simulink model "TD_THRUSTER_M0"  (R2019b)
settings: Solver=FixedStepAuto  StartTime=0.0  StopTime=10.0  RelTol=1e-3
undefined symbols (not defined in the file): w_neg_0, w_pos_0
settings Model: Creator=lbend  LastModifiedBy=peter
settings DebuggingCC: UnconnectedInputMsg=none  UnconnectedOutputMsg=none  UnconnectedLineMsg=none  SFMachineParentedDataDiag=error
settings ModelReferenceCC: EnableRefExpFcnMdlSchedulingChecks=off
settings RTWCC: Description=Generic Real-Time Target

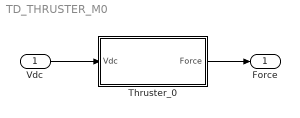
== system TD_THRUSTER_M0 ==
  Vdc : Inport
  Thruster_0 : Subsystem
  Force : Outport
  wires:
  Vdc/1 -> Thruster_0/1(Vdc)
  Thruster_0/1(Force) -> Force/1

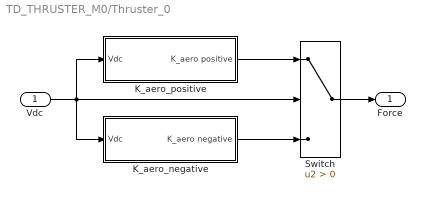
== system TD_THRUSTER_M0/Thruster_0 ==
  Vdc : Inport
  K_aero_negative : Subsystem
  K_aero_positive : Subsystem
  Switch : Switch  Criteria=u2 > Threshold
  Force : Outport
  wires:
  Switch/1 -> Force/1
  K_aero_positive/1(K_aero positive) -> Switch/1
  Vdc/1 -> K_aero_positive/1(Vdc), K_aero_negative/1(Vdc), Switch/2
  K_aero_negative/1(K_aero negative) -> Switch/3

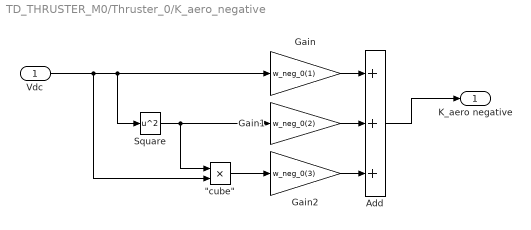
== system TD_THRUSTER_M0/Thruster_0/K_aero_negative ==
  Vdc : Inport
  "\"cube\"" : Product  Inputs=**
  Add : Sum  Inputs=+++
  Gain : Gain  Gain=w_neg_0(1)
  Gain1 : Gain  Gain=w_neg_0(2)
  Gain2 : Gain  Gain=w_neg_0(3)
  Square : Math  Operator=square  SignedPower=off  SaturateOnIntegerOverflow=on
  K_aero negative : Outport
  wires:
  Vdc/1 -> "\"cube\""/2, Square/1, Gain/1
  Gain/1 -> Add/1
  Square/1 -> "\"cube\""/1, Gain1/1
  Gain1/1 -> Add/2
  Gain2/1 -> Add/3
  "\"cube\""/1 -> Gain2/1
  Add/1 -> K_aero negative/1

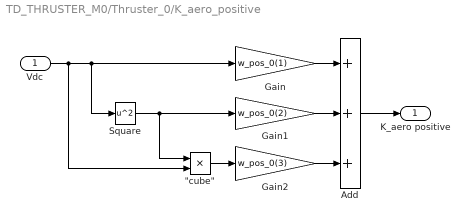
== system TD_THRUSTER_M0/Thruster_0/K_aero_positive ==
  Vdc : Inport
  "\"cube\"" : Product  Inputs=**
  Add : Sum  Inputs=+++
  Gain : Gain  Gain=w_pos_0(1)
  Gain1 : Gain  Gain=w_pos_0(2)
  Gain2 : Gain  Gain=w_pos_0(3)
  Square : Math  Operator=square  SignedPower=off  SaturateOnIntegerOverflow=on
  K_aero positive : Outport
  wires:
  Vdc/1 -> Gain/1, Square/1, "\"cube\""/2
  Add/1 -> K_aero positive/1
  Gain/1 -> Add/1
  Square/1 -> "\"cube\""/1, Gain1/1
  Gain1/1 -> Add/2
  "\"cube\""/1 -> Gain2/1
  Gain2/1 -> Add/3
